simulink model "simF16"  (Simulink 5.0)
settings: Solver=ode4  StartTime=0  StopTime=15  FixedStep=0.005  RelTol=1e-3
values from neighbouring files (symbols this model uses):
  control_trim = u0    [find_trim.m]    (also in find_trim_rev.m)
settings Model: Creator=keviczky  LastModifiedBy=Administrator  ExtModeAutoUpdateStatusClock=off  Decimation=50  LimitDataPoints=off  BooleanDataType=off

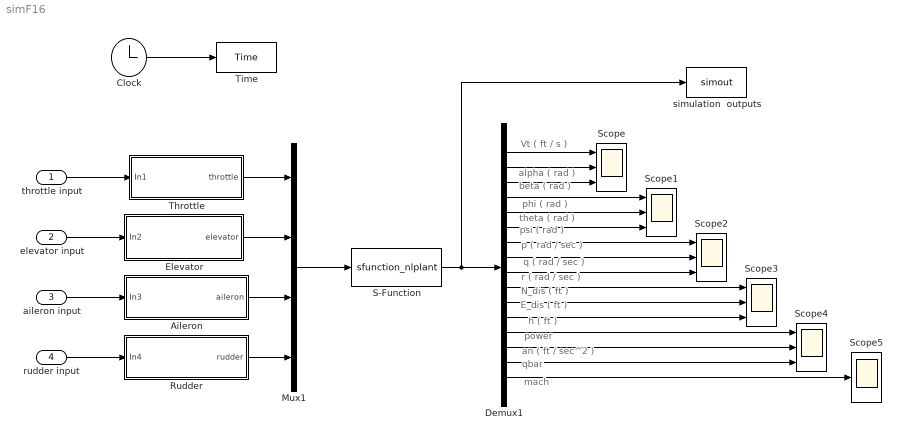
== system simF16 ==
  note: Vt ( ft / s )
  note: alpha ( rad )
  note: beta ( rad )
  note: phi ( rad )
  note: theta ( rad )
  note: psi ( rad )
  note: p ( rad / sec )
  note: q ( rad / sec )
  note: r ( rad / sec )
  note: N_dis ( ft )
  note: E_dis ( ft )
  note: h ( ft )
  note: power
  note: an ( ft / sec^2 )
  note: qbar
  note: mach
  throttle input : Inport
  elevator input : Inport  Port=2
  aileron input : Inport  Port=3
  rudder input : Inport  Port=4
  Aileron : Subsystem
  Clock : Clock
      settings: Decimation=50
  Demux1 : Demux  Outputs=16
  Elevator : Subsystem
  Mux1 : Mux
  Rudder : Subsystem
  S-Function : S-Function  FunctionName=sfunction_nlplant  Parameters="state_trim,  xcg"
  Scope{,1..4} (5 alike) : Scope  NumInputPorts=3
      Scope settings: YMin=600~0.0488613~-3.5e-014  YMax=600~0.0488613~-2.85e-014  SaveName=ScopeData6  Decimation=20
      Scope1 settings: TimeRange=10  YMin=0.126~3.2103~-0.32  YMax=0.143~3.21105~-0.245  SaveName=ScopeData7  Decimation=20
      Scope2 settings: YMin=-1.5e-006~-0.00075~-2.5e-006  YMax=1.5e-006~0.001~3e-006  SaveName=ScopeData8  Decimation=20
      Scope3 settings: YMin=-5~-5~-5  YMax=5~5~5  SaveName=ScopeData9  Decimation=20
      Scope4 settings: YMin=8.99847~0.999319~284.609  YMax=8.99853~0.99932~314.567  Decimation=20
  Scope5 : Scope
      settings: YMin=0.459181  YMax=0.459182
  Throttle : Subsystem
  Time : ToWorkspace  VariableName=Time  SampleTime=-1  SaveFormat=Array
      settings: Decimation=100
  simulation  outputs : ToWorkspace  VariableName=simout  SampleTime=-1  SaveFormat=Array
      settings: Decimation=100
  wires:
  S-Function/1 -> Demux1/1, simulation  outputs/1
  Clock/1 -> Time/1
  Demux1/1 -> Scope/1
  Demux1/2 -> Scope/2
  Demux1/3 -> Scope/3
  Demux1/5 -> Scope1/2
  Demux1/6 -> Scope1/3
  Demux1/7 -> Scope2/1
  Demux1/8 -> Scope2/2
  Demux1/9 -> Scope2/3
  Demux1/10 -> Scope3/1
  Demux1/11 -> Scope3/2
  Demux1/12 -> Scope3/3
  Demux1/13 -> Scope4/1
  Demux1/14 -> Scope4/2
  Demux1/4 -> Scope1/1
  Demux1/15 -> Scope4/3
  Demux1/16 -> Scope5/1
  Throttle/1(throttle) -> Mux1/1
  Mux1/1 -> S-Function/1
  throttle input/1 -> Throttle/1(In1)
  elevator input/1 -> Elevator/1(In2)
  aileron input/1 -> Aileron/1(In3)
  rudder input/1 -> Rudder/1(In4)
  Elevator/1(elevator) -> Mux1/2
  Aileron/1(aileron) -> Mux1/3
  Rudder/1(rudder) -> Mux1/4

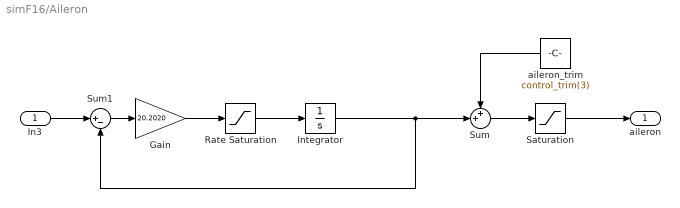
== system simF16/Aileron ==
  In3 : Inport
  Gain : Gain  Gain=20.2020  SaturateOnIntegerOverflow=on
  Integrator : Integrator  UpperSaturationLimit=21.5  LowerSaturationLimit=-21.5
  Rate Saturation : Saturate  UpperLimit=80  LowerLimit=-80
  Saturation : Saturate  UpperLimit=21.5  LowerLimit=-21.5
  Sum : Sum  Inputs=++|  SaturateOnIntegerOverflow=on  InputSameDT=on
  Sum1 : Sum  Inputs=|+-  SaturateOnIntegerOverflow=on  InputSameDT=on
  aileron_trim : Constant  Orientation=left  Value=control_trim(3)
  aileron : Outport
  wires:
  In3/1 -> Sum1/1
  Sum1/1 -> Gain/1
  Gain/1 -> Rate Saturation/1
  Rate Saturation/1 -> Integrator/1
  Integrator/1 -> Sum1/2, Sum/2
  Sum/1 -> Saturation/1
  aileron_trim/1 -> Sum/1
  Saturation/1 -> aileron/1

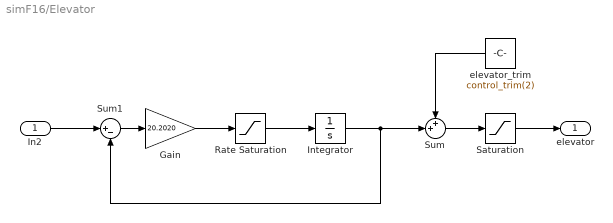
== system simF16/Elevator ==
  In2 : Inport
  Gain : Gain  Gain=20.2020  SaturateOnIntegerOverflow=on
  Integrator : Integrator  UpperSaturationLimit=25  LowerSaturationLimit=-25
  Rate Saturation : Saturate  UpperLimit=60  LowerLimit=-60
  Saturation : Saturate  UpperLimit=25  LowerLimit=-25
  Sum : Sum  Inputs=++|  SaturateOnIntegerOverflow=on  InputSameDT=on
  Sum1 : Sum  Inputs=|+-  SaturateOnIntegerOverflow=on  InputSameDT=on
  elevator_trim : Constant  Orientation=left  Value=control_trim(2)
  elevator : Outport
  wires:
  In2/1 -> Sum1/1
  Sum1/1 -> Gain/1
  Gain/1 -> Rate Saturation/1
  Rate Saturation/1 -> Integrator/1
  Integrator/1 -> Sum1/2, Sum/2
  Sum/1 -> Saturation/1
  elevator_trim/1 -> Sum/1
  Saturation/1 -> elevator/1

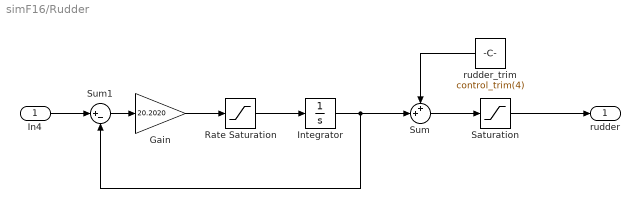
== system simF16/Rudder ==
  In4 : Inport
  Gain : Gain  Gain=20.2020  SaturateOnIntegerOverflow=on
  Integrator : Integrator  UpperSaturationLimit=30  LowerSaturationLimit=-30
  Rate Saturation : Saturate  UpperLimit=120  LowerLimit=-120
  Saturation : Saturate  UpperLimit=30  LowerLimit=-30
  Sum : Sum  Inputs=++|  SaturateOnIntegerOverflow=on  InputSameDT=on
  Sum1 : Sum  Inputs=|+-  SaturateOnIntegerOverflow=on  InputSameDT=on
  rudder_trim : Constant  Orientation=left  Value=control_trim(4)
  rudder : Outport
  wires:
  In4/1 -> Sum1/1
  Sum1/1 -> Gain/1
  Gain/1 -> Rate Saturation/1
  Rate Saturation/1 -> Integrator/1
  Integrator/1 -> Sum1/2, Sum/2
  Saturation/1 -> rudder/1
  Sum/1 -> Saturation/1
  rudder_trim/1 -> Sum/1

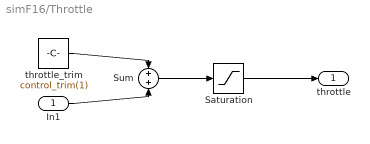
== system simF16/Throttle ==
  In1 : Inport
  Saturation : Saturate  UpperLimit=1  LowerLimit=0
  Sum : Sum  SaturateOnIntegerOverflow=on  InputSameDT=on
  throttle_trim : Constant  Value=control_trim(1)
  throttle : Outport
  wires:
  throttle_trim/1 -> Sum/1
  In1/1 -> Sum/2
  Sum/1 -> Saturation/1
  Saturation/1 -> throttle/1
